simulink model "ADU_Integration_R2014a_simulation"  (R2014a)
settings: Solver=FixedStepDiscrete  StartTime=285  StopTime=300  FixedStep=0.01  RelTol=1e-3
PostLoadFcn:
  | , if any(exist('dsrtsu_mdlpostloadfcn', 'file') == [2, 3, 6]), try dsrtsu_mdlpostloadfcn('Execute', bdroot); catch fprintf('Error in PostLoadFcn (dsrtsu_mdlpostloadfcn) for model "%s":\n %s\n', bdroot, lasterr); end, end,
InitFcn:
  | load 'data/chi2_dat';
  | load 'data/Line_struct';
  | load 'data/innerLNM_1';
  | load 'data/middleLNM_2';
  | load 'data/outerLNM_1';
  | load 'data/landmarks_patac_schimmel_ccw';
  | load 'data/patac_navi_array';
  | load 'data/sensor';
  | load 'data/map_struct';
  | addpath map_src
  | Integration_Parameter;
  | load 'TestData_001';
values from neighbouring files (symbols this model uses):
  TestData_001 =     [TestData_001.mat]
undefined symbols (not defined in the file or in its folder): chi2_dat, innerLNM_1, landmarks_patac_schimmel_ccw, middleLNM_2, outerLNM_1, patac_navi_array
libraries: simulink x36, rtican x1
(part 4 of 22)

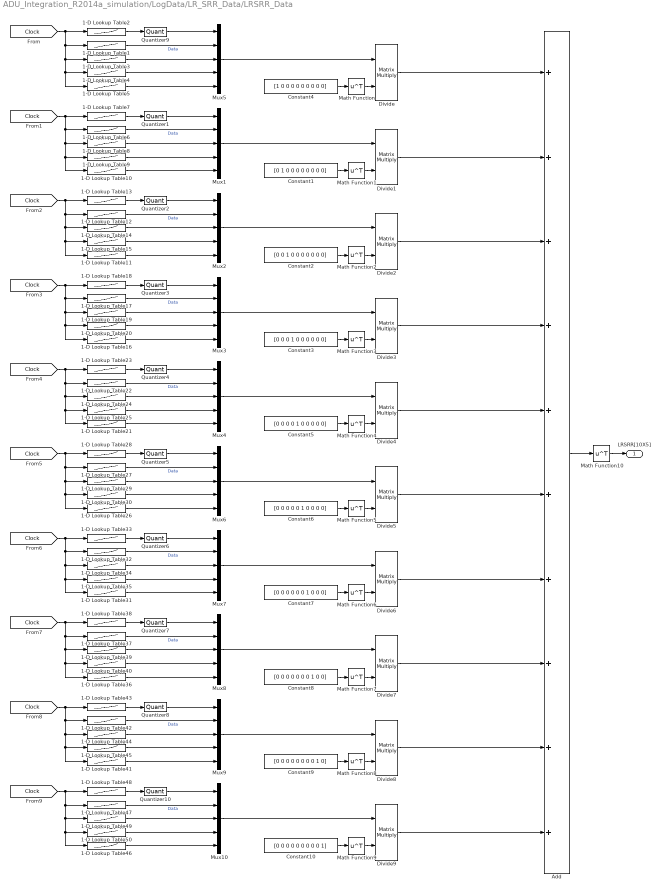
== system ADU_Integration_R2014a_simulation/LogData/LR_SRR_Data/LRSRR_Data ==
  1-D Lookup Table1 : Lookup_n-D  NumberOfTableDimensions=1  BreakpointsForDimension1=TestData_001.X.Data  Table=TestData_001.Y(StartNum+1+5*0).Data  RndMeth=Simplest  InputSameDT=on
  1-D Lookup Table10 : Lookup_n-D  NumberOfTableDimensions=1  BreakpointsForDimension1=TestData_001.X.Data  Table=TestData_001.Y(StartNum+4+5*1).Data  RndMeth=Simplest  InputSameDT=on
  1-D Lookup Table11 : Lookup_n-D  NumberOfTableDimensions=1  BreakpointsForDimension1=TestData_001.X.Data  Table=TestData_001.Y(StartNum+4+5*2).Data  RndMeth=Simplest  InputSameDT=on
  1-D Lookup Table12 : Lookup_n-D  NumberOfTableDimensions=1  BreakpointsForDimension1=TestData_001.X.Data  Table=TestData_001.Y(StartNum+1+5*2).Data  RndMeth=Simplest  InputSameDT=on
  1-D Lookup Table13 : Lookup_n-D  NumberOfTableDimensions=1  BreakpointsForDimension1=TestData_001.X.Data  Table=TestData_001.Y(StartNum+5*2).Data  RndMeth=Simplest  InputSameDT=on
  1-D Lookup Table14 : Lookup_n-D  NumberOfTableDimensions=1  BreakpointsForDimension1=TestData_001.X.Data  Table=TestData_001.Y(StartNum+2+5*2).Data  RndMeth=Simplest  InputSameDT=on
  1-D Lookup Table15 : Lookup_n-D  NumberOfTableDimensions=1  BreakpointsForDimension1=TestData_001.X.Data  Table=TestData_001.Y(StartNum+3+5*2).Data  RndMeth=Simplest  InputSameDT=on
  1-D Lookup Table16 : Lookup_n-D  NumberOfTableDimensions=1  BreakpointsForDimension1=TestData_001.X.Data  Table=TestData_001.Y(StartNum+4+5*3).Data  RndMeth=Simplest  InputSameDT=on
  1-D Lookup Table17 : Lookup_n-D  NumberOfTableDimensions=1  BreakpointsForDimension1=TestData_001.X.Data  Table=TestData_001.Y(StartNum+1+5*3).Data  RndMeth=Simplest  InputSameDT=on
  1-D Lookup Table18 : Lookup_n-D  NumberOfTableDimensions=1  BreakpointsForDimension1=TestData_001.X.Data  Table=TestData_001.Y(StartNum+5*3).Data  RndMeth=Simplest  InputSameDT=on
  1-D Lookup Table19 : Lookup_n-D  NumberOfTableDimensions=1  BreakpointsForDimension1=TestData_001.X.Data  Table=TestData_001.Y(StartNum+2+5*3).Data  RndMeth=Simplest  InputSameDT=on
  1-D Lookup Table2 : Lookup_n-D  NumberOfTableDimensions=1  BreakpointsForDimension1=TestData_001.X.Data  Table=TestData_001.Y(StartNum+5*0).Data  RndMeth=Simplest  InputSameDT=on
  1-D Lookup Table20 : Lookup_n-D  NumberOfTableDimensions=1  BreakpointsForDimension1=TestData_001.X.Data  Table=TestData_001.Y(StartNum+3+5*3).Data  RndMeth=Simplest  InputSameDT=on
  1-D Lookup Table21 : Lookup_n-D  NumberOfTableDimensions=1  BreakpointsForDimension1=TestData_001.X.Data  Table=TestData_001.Y(StartNum+4+5*4).Data  RndMeth=Simplest  InputSameDT=on
  1-D Lookup Table22 : Lookup_n-D  NumberOfTableDimensions=1  BreakpointsForDimension1=TestData_001.X.Data  Table=TestData_001.Y(StartNum+1+5*4).Data  RndMeth=Simplest  InputSameDT=on
  1-D Lookup Table23 : Lookup_n-D  NumberOfTableDimensions=1  BreakpointsForDimension1=TestData_001.X.Data  Table=TestData_001.Y(StartNum+5*4).Data  RndMeth=Simplest  InputSameDT=on
  1-D Lookup Table24 : Lookup_n-D  NumberOfTableDimensions=1  BreakpointsForDimension1=TestData_001.X.Data  Table=TestData_001.Y(StartNum+2+5*4).Data  RndMeth=Simplest  InputSameDT=on
  1-D Lookup Table25 : Lookup_n-D  NumberOfTableDimensions=1  BreakpointsForDimension1=TestData_001.X.Data  Table=TestData_001.Y(StartNum+3+5*4).Data  RndMeth=Simplest  InputSameDT=on
  1-D Lookup Table26 : Lookup_n-D  NumberOfTableDimensions=1  BreakpointsForDimension1=TestData_001.X.Data  Table=TestData_001.Y(StartNum+4+5*5).Data  RndMeth=Simplest  InputSameDT=on
  1-D Lookup Table27 : Lookup_n-D  NumberOfTableDimensions=1  BreakpointsForDimension1=TestData_001.X.Data  Table=TestData_001.Y(StartNum+1+5*5).Data  RndMeth=Simplest  InputSameDT=on
  1-D Lookup Table28 : Lookup_n-D  NumberOfTableDimensions=1  BreakpointsForDimension1=TestData_001.X.Data  Table=TestData_001.Y(StartNum+5*5).Data  RndMeth=Simplest  InputSameDT=on
  1-D Lookup Table29 : Lookup_n-D  NumberOfTableDimensions=1  BreakpointsForDimension1=TestData_001.X.Data  Table=TestData_001.Y(StartNum+2+5*5).Data  RndMeth=Simplest  InputSameDT=on
  1-D Lookup Table3 : Lookup_n-D  NumberOfTableDimensions=1  BreakpointsForDimension1=TestData_001.X.Data  Table=TestData_001.Y(StartNum+2+5*0).Data  RndMeth=Simplest  InputSameDT=on
  1-D Lookup Table30 : Lookup_n-D  NumberOfTableDimensions=1  BreakpointsForDimension1=TestData_001.X.Data  Table=TestData_001.Y(StartNum+3+5*5).Data  RndMeth=Simplest  InputSameDT=on
  1-D Lookup Table31 : Lookup_n-D  NumberOfTableDimensions=1  BreakpointsForDimension1=TestData_001.X.Data  Table=TestData_001.Y(StartNum+4+5*6).Data  RndMeth=Simplest  InputSameDT=on
  1-D Lookup Table32 : Lookup_n-D  NumberOfTableDimensions=1  BreakpointsForDimension1=TestData_001.X.Data  Table=TestData_001.Y(StartNum+1+5*6).Data  RndMeth=Simplest  InputSameDT=on
  1-D Lookup Table33 : Lookup_n-D  NumberOfTableDimensions=1  BreakpointsForDimension1=TestData_001.X.Data  Table=TestData_001.Y(StartNum+5*6).Data  RndMeth=Simplest  InputSameDT=on
  1-D Lookup Table34 : Lookup_n-D  NumberOfTableDimensions=1  BreakpointsForDimension1=TestData_001.X.Data  Table=TestData_001.Y(StartNum+2+5*6).Data  RndMeth=Simplest  InputSameDT=on
  1-D Lookup Table35 : Lookup_n-D  NumberOfTableDimensions=1  BreakpointsForDimension1=TestData_001.X.Data  Table=TestData_001.Y(StartNum+3+5*6).Data  RndMeth=Simplest  InputSameDT=on
  1-D Lookup Table36 : Lookup_n-D  NumberOfTableDimensions=1  BreakpointsForDimension1=TestData_001.X.Data  Table=TestData_001.Y(StartNum+4+5*7).Data  RndMeth=Simplest  InputSameDT=on
  1-D Lookup Table37 : Lookup_n-D  NumberOfTableDimensions=1  BreakpointsForDimension1=TestData_001.X.Data  Table=TestData_001.Y(StartNum+1+5*7).Data  RndMeth=Simplest  InputSameDT=on
  1-D Lookup Table38 : Lookup_n-D  NumberOfTableDimensions=1  BreakpointsForDimension1=TestData_001.X.Data  Table=TestData_001.Y(StartNum+5*7).Data  RndMeth=Simplest  InputSameDT=on
  1-D Lookup Table39 : Lookup_n-D  NumberOfTableDimensions=1  BreakpointsForDimension1=TestData_001.X.Data  Table=TestData_001.Y(StartNum+2+5*7).Data  RndMeth=Simplest  InputSameDT=on
  1-D Lookup Table4 : Lookup_n-D  NumberOfTableDimensions=1  BreakpointsForDimension1=TestData_001.X.Data  Table=TestData_001.Y(StartNum+3+5*0).Data  RndMeth=Simplest  InputSameDT=on
  1-D Lookup Table40 : Lookup_n-D  NumberOfTableDimensions=1  BreakpointsForDimension1=TestData_001.X.Data  Table=TestData_001.Y(StartNum+3+5*7).Data  RndMeth=Simplest  InputSameDT=on
  1-D Lookup Table41 : Lookup_n-D  NumberOfTableDimensions=1  BreakpointsForDimension1=TestData_001.X.Data  Table=TestData_001.Y(StartNum+4+5*8).Data  RndMeth=Simplest  InputSameDT=on
  1-D Lookup Table42 : Lookup_n-D  NumberOfTableDimensions=1  BreakpointsForDimension1=TestData_001.X.Data  Table=TestData_001.Y(StartNum+1+5*8).Data  RndMeth=Simplest  InputSameDT=on
  1-D Lookup Table43 : Lookup_n-D  NumberOfTableDimensions=1  BreakpointsForDimension1=TestData_001.X.Data  Table=TestData_001.Y(StartNum+5*8).Data  RndMeth=Simplest  InputSameDT=on
  1-D Lookup Table44 : Lookup_n-D  NumberOfTableDimensions=1  BreakpointsForDimension1=TestData_001.X.Data  Table=TestData_001.Y(StartNum+2+5*8).Data  RndMeth=Simplest  InputSameDT=on
  1-D Lookup Table45 : Lookup_n-D  NumberOfTableDimensions=1  BreakpointsForDimension1=TestData_001.X.Data  Table=TestData_001.Y(StartNum+3+5*8).Data  RndMeth=Simplest  InputSameDT=on
  1-D Lookup Table46 : Lookup_n-D  NumberOfTableDimensions=1  BreakpointsForDimension1=TestData_001.X.Data  Table=TestData_001.Y(StartNum+4+5*9).Data  RndMeth=Simplest  InputSameDT=on
  1-D Lookup Table47 : Lookup_n-D  NumberOfTableDimensions=1  BreakpointsForDimension1=TestData_001.X.Data  Table=TestData_001.Y(StartNum+1+5*9).Data  RndMeth=Simplest  InputSameDT=on
  1-D Lookup Table48 : Lookup_n-D  NumberOfTableDimensions=1  BreakpointsForDimension1=TestData_001.X.Data  Table=TestData_001.Y(StartNum+5*9).Data  RndMeth=Simplest  InputSameDT=on
  1-D Lookup Table49 : Lookup_n-D  NumberOfTableDimensions=1  BreakpointsForDimension1=TestData_001.X.Data  Table=TestData_001.Y(StartNum+2+5*9).Data  RndMeth=Simplest  InputSameDT=on
  1-D Lookup Table5 : Lookup_n-D  NumberOfTableDimensions=1  BreakpointsForDimension1=TestData_001.X.Data  Table=TestData_001.Y(StartNum+4+5*0).Data  RndMeth=Simplest  InputSameDT=on
  1-D Lookup Table50 : Lookup_n-D  NumberOfTableDimensions=1  BreakpointsForDimension1=TestData_001.X.Data  Table=TestData_001.Y(StartNum+3+5*9).Data  RndMeth=Simplest  InputSameDT=on
  1-D Lookup Table6 : Lookup_n-D  NumberOfTableDimensions=1  BreakpointsForDimension1=TestData_001.X.Data  Table=TestData_001.Y(StartNum+1+5*1).Data  RndMeth=Simplest  InputSameDT=on
  1-D Lookup Table7 : Lookup_n-D  NumberOfTableDimensions=1  BreakpointsForDimension1=TestData_001.X.Data  Table=TestData_001.Y(StartNum+5*1).Data  RndMeth=Simplest  InputSameDT=on
  1-D Lookup Table8 : Lookup_n-D  NumberOfTableDimensions=1  BreakpointsForDimension1=TestData_001.X.Data  Table=TestData_001.Y(StartNum+2+5*1).Data  RndMeth=Simplest  InputSameDT=on
  1-D Lookup Table9 : Lookup_n-D  NumberOfTableDimensions=1  BreakpointsForDimension1=TestData_001.X.Data  Table=TestData_001.Y(StartNum+3+5*1).Data  RndMeth=Simplest  InputSameDT=on
  Add : Sum  Inputs=++++++++++
  Constant1 : Constant  Value=[0 1 0 0 0 0 0 0 0 0]
  Constant10 : Constant  Value=[0 0 0 0 0 0 0 0 0 1]
  Constant2 : Constant  Value=[0 0 1 0 0 0 0 0 0 0]
  Constant3 : Constant  Value=[0 0 0 1 0 0 0 0 0 0]
  Constant4 : Constant  Value=[1 0 0 0 0 0 0 0 0 0]
  Constant5 : Constant  Value=[0 0 0 0 1 0 0 0 0 0]
  Constant6 : Constant  Value=[0 0 0 0 0 1 0 0 0 0]
  Constant7 : Constant  Value=[0 0 0 0 0 0 1 0 0 0]
  Constant8 : Constant  Value=[0 0 0 0 0 0 0 1 0 0]
  Constant9 : Constant  Value=[0 0 0 0 0 0 0 0 1 0]
  Divide{,1..9} (10 alike) : Product  Inputs=**  Multiplication=Matrix(*)
  Math Function{,1..10} (11 alike) : Math  Operator=transpose  SaturateOnIntegerOverflow=on
  Mux{1..10} (10 alike) : Mux  Inputs=5
  Quantizer{1..10} (10 alike) : Quantizer  QuantizationInterval=1
  LRSRR[10X5] : Outport
  wires:
  Mux5/1 -> Divide/1
  Constant4/1 -> Math Function/1
  Math Function/1 -> Divide/2
  Divide/1 -> Add/1
  Math Function4/1 -> Divide4/2
  Math Function3/1 -> Divide3/2
  Divide3/1 -> Add/4
  Constant9/1 -> Math Function8/1
  Math Function6/1 -> Divide6/2
  Divide1/1 -> Add/2
  Divide4/1 -> Add/5
  Quantizer9/1 -> Mux5/1
  Constant7/1 -> Math Function6/1
  Divide2/1 -> Add/3
  Divide9/1 -> Add/10
  Constant3/1 -> Math Function3/1
  Divide5/1 -> Add/6
  Math Function5/1 -> Divide5/2
  1-D Lookup Table4/1 -> Mux5/4
  1-D Lookup Table3/1 -> Mux5/3
  Constant8/1 -> Math Function7/1
  Divide6/1 -> Add/7
  Math Function8/1 -> Divide8/2
  Constant5/1 -> Math Function4/1
  Math Function9/1 -> Divide9/2
  Math Function7/1 -> Divide7/2
  Constant10/1 -> Math Function9/1
  Math Function2/1 -> Divide2/2
  Constant1/1 -> Math Function1/1
  Divide7/1 -> Add/8
  Divide8/1 -> Add/9
  Constant2/1 -> Math Function2/1
  Math Function1/1 -> Divide1/2
  Constant6/1 -> Math Function5/1
  Add/1 -> Math Function10/1
  Math Function10/1 -> LRSRR[10X5]/1
  1-D Lookup Table2/1 -> Quantizer9/1
  [Clock] -> 1-D Lookup Table2/1, 1-D Lookup Table1/1, 1-D Lookup Table5/1, 1-D Lookup Table4/1, 1-D Lookup Table3/1
  1-D Lookup Table1/1 -> Mux5/2  "Data"
  1-D Lookup Table5/1 -> Mux5/5
  Mux1/1 -> Divide1/1
  Quantizer1/1 -> Mux1/1
  1-D Lookup Table9/1 -> Mux1/4
  1-D Lookup Table8/1 -> Mux1/3
  1-D Lookup Table7/1 -> Quantizer1/1
  [Clock] -> 1-D Lookup Table7/1, 1-D Lookup Table6/1, 1-D Lookup Table8/1, 1-D Lookup Table10/1, 1-D Lookup Table9/1
  1-D Lookup Table6/1 -> Mux1/2  "Data"
  1-D Lookup Table10/1 -> Mux1/5
  Mux2/1 -> Divide2/1
  Quantizer2/1 -> Mux2/1
  1-D Lookup Table15/1 -> Mux2/4
  1-D Lookup Table14/1 -> Mux2/3
  1-D Lookup Table13/1 -> Quantizer2/1
  [Clock] -> 1-D Lookup Table13/1, 1-D Lookup Table12/1, 1-D Lookup Table14/1, 1-D Lookup Table15/1, 1-D Lookup Table11/1
  1-D Lookup Table12/1 -> Mux2/2  "Data"
  1-D Lookup Table11/1 -> Mux2/5
  Mux3/1 -> Divide3/1
  Quantizer3/1 -> Mux3/1
  1-D Lookup Table20/1 -> Mux3/4
  1-D Lookup Table19/1 -> Mux3/3
  1-D Lookup Table18/1 -> Quantizer3/1
  [Clock] -> 1-D Lookup Table18/1, 1-D Lookup Table17/1, 1-D Lookup Table19/1, 1-D Lookup Table20/1, 1-D Lookup Table16/1
  1-D Lookup Table17/1 -> Mux3/2  "Data"
  1-D Lookup Table16/1 -> Mux3/5
  Mux4/1 -> Divide4/1
  Quantizer4/1 -> Mux4/1
  1-D Lookup Table25/1 -> Mux4/4
  1-D Lookup Table24/1 -> Mux4/3
  1-D Lookup Table23/1 -> Quantizer4/1
  [Clock] -> 1-D Lookup Table23/1, 1-D Lookup Table22/1, 1-D Lookup Table24/1, 1-D Lookup Table21/1, 1-D Lookup Table25/1
  1-D Lookup Table22/1 -> Mux4/2  "Data"
  1-D Lookup Table21/1 -> Mux4/5
  Mux6/1 -> Divide5/1
  Quantizer5/1 -> Mux6/1
  1-D Lookup Table30/1 -> Mux6/4
  1-D Lookup Table29/1 -> Mux6/3
  1-D Lookup Table28/1 -> Quantizer5/1
  [Clock] -> 1-D Lookup Table28/1, 1-D Lookup Table27/1, 1-D Lookup Table29/1, 1-D Lookup Table30/1, 1-D Lookup Table26/1
  1-D Lookup Table27/1 -> Mux6/2  "Data"
  1-D Lookup Table26/1 -> Mux6/5
  Mux7/1 -> Divide6/1
  Quantizer6/1 -> Mux7/1
  1-D Lookup Table35/1 -> Mux7/4
  1-D Lookup Table34/1 -> Mux7/3
  1-D Lookup Table33/1 -> Quantizer6/1
  [Clock] -> 1-D Lookup Table33/1, 1-D Lookup Table32/1, 1-D Lookup Table34/1, 1-D Lookup Table31/1, 1-D Lookup Table35/1
  1-D Lookup Table32/1 -> Mux7/2  "Data"
  1-D Lookup Table31/1 -> Mux7/5
  Mux8/1 -> Divide7/1
  Quantizer7/1 -> Mux8/1
  1-D Lookup Table40/1 -> Mux8/4
  1-D Lookup Table39/1 -> Mux8/3
  1-D Lookup Table38/1 -> Quantizer7/1
  [Clock] -> 1-D Lookup Table38/1, 1-D Lookup Table37/1, 1-D Lookup Table39/1, 1-D Lookup Table40/1, 1-D Lookup Table36/1
  1-D Lookup Table37/1 -> Mux8/2  "Data"
  1-D Lookup Table36/1 -> Mux8/5
  Mux9/1 -> Divide8/1
  Quantizer8/1 -> Mux9/1
  1-D Lookup Table45/1 -> Mux9/4
  1-D Lookup Table44/1 -> Mux9/3
  1-D Lookup Table43/1 -> Quantizer8/1
  [Clock] -> 1-D Lookup Table43/1, 1-D Lookup Table42/1, 1-D Lookup Table44/1, 1-D Lookup Table41/1, 1-D Lookup Table45/1
  1-D Lookup Table42/1 -> Mux9/2  "Data"
  1-D Lookup Table41/1 -> Mux9/5
  Mux10/1 -> Divide9/1
  Quantizer10/1 -> Mux10/1
  1-D Lookup Table50/1 -> Mux10/4
  1-D Lookup Table49/1 -> Mux10/3
  1-D Lookup Table48/1 -> Quantizer10/1
  [Clock] -> 1-D Lookup Table48/1, 1-D Lookup Table47/1, 1-D Lookup Table49/1, 1-D Lookup Table50/1, 1-D Lookup Table46/1
  1-D Lookup Table47/1 -> Mux10/2  "Data"
  1-D Lookup Table46/1 -> Mux10/5

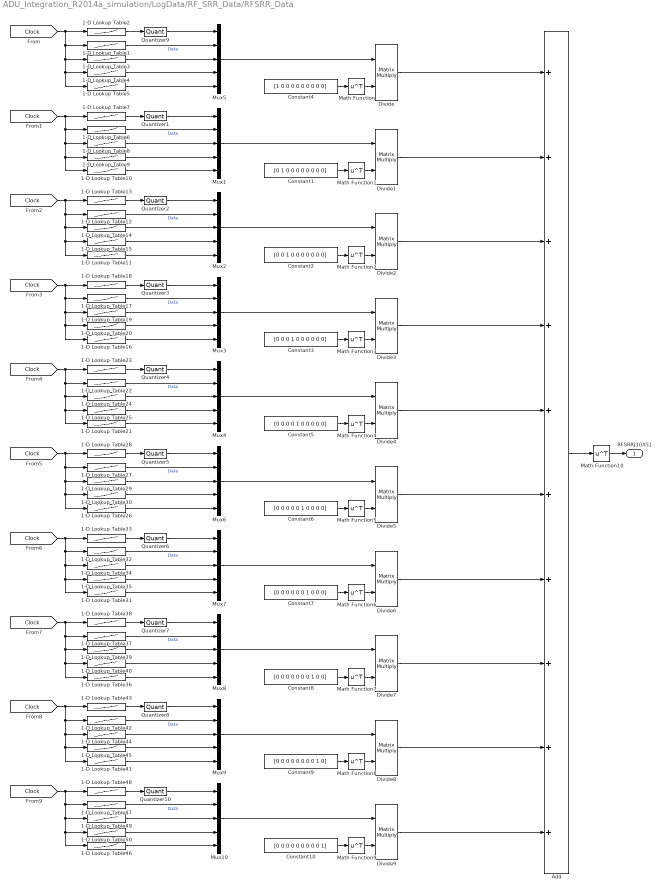
== system ADU_Integration_R2014a_simulation/LogData/RF_SRR_Data/RFSRR_Data ==
  1-D Lookup Table1 : Lookup_n-D  NumberOfTableDimensions=1  BreakpointsForDimension1=TestData_001.X.Data  Table=TestData_001.Y(StartNum+1+5*0).Data  RndMeth=Simplest  InputSameDT=on
  1-D Lookup Table10 : Lookup_n-D  NumberOfTableDimensions=1  BreakpointsForDimension1=TestData_001.X.Data  Table=TestData_001.Y(StartNum+4+5*1).Data  RndMeth=Simplest  InputSameDT=on
  1-D Lookup Table11 : Lookup_n-D  NumberOfTableDimensions=1  BreakpointsForDimension1=TestData_001.X.Data  Table=TestData_001.Y(StartNum+4+5*2).Data  RndMeth=Simplest  InputSameDT=on
  1-D Lookup Table12 : Lookup_n-D  NumberOfTableDimensions=1  BreakpointsForDimension1=TestData_001.X.Data  Table=TestData_001.Y(StartNum+1+5*2).Data  RndMeth=Simplest  InputSameDT=on
  1-D Lookup Table13 : Lookup_n-D  NumberOfTableDimensions=1  BreakpointsForDimension1=TestData_001.X.Data  Table=TestData_001.Y(StartNum+5*2).Data  RndMeth=Simplest  InputSameDT=on
  1-D Lookup Table14 : Lookup_n-D  NumberOfTableDimensions=1  BreakpointsForDimension1=TestData_001.X.Data  Table=TestData_001.Y(StartNum+2+5*2).Data  RndMeth=Simplest  InputSameDT=on
  1-D Lookup Table15 : Lookup_n-D  NumberOfTableDimensions=1  BreakpointsForDimension1=TestData_001.X.Data  Table=TestData_001.Y(StartNum+3+5*2).Data  RndMeth=Simplest  InputSameDT=on
  1-D Lookup Table16 : Lookup_n-D  NumberOfTableDimensions=1  BreakpointsForDimension1=TestData_001.X.Data  Table=TestData_001.Y(StartNum+4+5*3).Data  RndMeth=Simplest  InputSameDT=on
  1-D Lookup Table17 : Lookup_n-D  NumberOfTableDimensions=1  BreakpointsForDimension1=TestData_001.X.Data  Table=TestData_001.Y(StartNum+1+5*3).Data  RndMeth=Simplest  InputSameDT=on
  1-D Lookup Table18 : Lookup_n-D  NumberOfTableDimensions=1  BreakpointsForDimension1=TestData_001.X.Data  Table=TestData_001.Y(StartNum+5*3).Data  RndMeth=Simplest  InputSameDT=on
  1-D Lookup Table19 : Lookup_n-D  NumberOfTableDimensions=1  BreakpointsForDimension1=TestData_001.X.Data  Table=TestData_001.Y(StartNum+2+5*3).Data  RndMeth=Simplest  InputSameDT=on
  1-D Lookup Table2 : Lookup_n-D  NumberOfTableDimensions=1  BreakpointsForDimension1=TestData_001.X.Data  Table=TestData_001.Y(StartNum+5*0).Data  RndMeth=Simplest  InputSameDT=on
  1-D Lookup Table20 : Lookup_n-D  NumberOfTableDimensions=1  BreakpointsForDimension1=TestData_001.X.Data  Table=TestData_001.Y(StartNum+3+5*3).Data  RndMeth=Simplest  InputSameDT=on
  1-D Lookup Table21 : Lookup_n-D  NumberOfTableDimensions=1  BreakpointsForDimension1=TestData_001.X.Data  Table=TestData_001.Y(StartNum+4+5*4).Data  RndMeth=Simplest  InputSameDT=on
  1-D Lookup Table22 : Lookup_n-D  NumberOfTableDimensions=1  BreakpointsForDimension1=TestData_001.X.Data  Table=TestData_001.Y(StartNum+1+5*4).Data  RndMeth=Simplest  InputSameDT=on
  1-D Lookup Table23 : Lookup_n-D  NumberOfTableDimensions=1  BreakpointsForDimension1=TestData_001.X.Data  Table=TestData_001.Y(StartNum+5*4).Data  RndMeth=Simplest  InputSameDT=on
  1-D Lookup Table24 : Lookup_n-D  NumberOfTableDimensions=1  BreakpointsForDimension1=TestData_001.X.Data  Table=TestData_001.Y(StartNum+2+5*4).Data  RndMeth=Simplest  InputSameDT=on
  1-D Lookup Table25 : Lookup_n-D  NumberOfTableDimensions=1  BreakpointsForDimension1=TestData_001.X.Data  Table=TestData_001.Y(StartNum+3+5*4).Data  RndMeth=Simplest  InputSameDT=on
  1-D Lookup Table26 : Lookup_n-D  NumberOfTableDimensions=1  BreakpointsForDimension1=TestData_001.X.Data  Table=TestData_001.Y(StartNum+4+5*5).Data  RndMeth=Simplest  InputSameDT=on
  1-D Lookup Table27 : Lookup_n-D  NumberOfTableDimensions=1  BreakpointsForDimension1=TestData_001.X.Data  Table=TestData_001.Y(StartNum+1+5*5).Data  RndMeth=Simplest  InputSameDT=on
  1-D Lookup Table28 : Lookup_n-D  NumberOfTableDimensions=1  BreakpointsForDimension1=TestData_001.X.Data  Table=TestData_001.Y(StartNum+5*5).Data  RndMeth=Simplest  InputSameDT=on
  1-D Lookup Table29 : Lookup_n-D  NumberOfTableDimensions=1  BreakpointsForDimension1=TestData_001.X.Data  Table=TestData_001.Y(StartNum+2+5*5).Data  RndMeth=Simplest  InputSameDT=on
  1-D Lookup Table3 : Lookup_n-D  NumberOfTableDimensions=1  BreakpointsForDimension1=TestData_001.X.Data  Table=TestData_001.Y(StartNum+2+5*0).Data  RndMeth=Simplest  InputSameDT=on
  1-D Lookup Table30 : Lookup_n-D  NumberOfTableDimensions=1  BreakpointsForDimension1=TestData_001.X.Data  Table=TestData_001.Y(StartNum+3+5*5).Data  RndMeth=Simplest  InputSameDT=on
  1-D Lookup Table31 : Lookup_n-D  NumberOfTableDimensions=1  BreakpointsForDimension1=TestData_001.X.Data  Table=TestData_001.Y(StartNum+4+5*6).Data  RndMeth=Simplest  InputSameDT=on
  1-D Lookup Table32 : Lookup_n-D  NumberOfTableDimensions=1  BreakpointsForDimension1=TestData_001.X.Data  Table=TestData_001.Y(StartNum+1+5*6).Data  RndMeth=Simplest  InputSameDT=on
  1-D Lookup Table33 : Lookup_n-D  NumberOfTableDimensions=1  BreakpointsForDimension1=TestData_001.X.Data  Table=TestData_001.Y(StartNum+5*6).Data  RndMeth=Simplest  InputSameDT=on
  1-D Lookup Table34 : Lookup_n-D  NumberOfTableDimensions=1  BreakpointsForDimension1=TestData_001.X.Data  Table=TestData_001.Y(StartNum+2+5*6).Data  RndMeth=Simplest  InputSameDT=on
  1-D Lookup Table35 : Lookup_n-D  NumberOfTableDimensions=1  BreakpointsForDimension1=TestData_001.X.Data  Table=TestData_001.Y(StartNum+3+5*6).Data  RndMeth=Simplest  InputSameDT=on
  1-D Lookup Table36 : Lookup_n-D  NumberOfTableDimensions=1  BreakpointsForDimension1=TestData_001.X.Data  Table=TestData_001.Y(StartNum+4+5*7).Data  RndMeth=Simplest  InputSameDT=on
  1-D Lookup Table37 : Lookup_n-D  NumberOfTableDimensions=1  BreakpointsForDimension1=TestData_001.X.Data  Table=TestData_001.Y(StartNum+1+5*7).Data  RndMeth=Simplest  InputSameDT=on
  1-D Lookup Table38 : Lookup_n-D  NumberOfTableDimensions=1  BreakpointsForDimension1=TestData_001.X.Data  Table=TestData_001.Y(StartNum+5*7).Data  RndMeth=Simplest  InputSameDT=on
  1-D Lookup Table39 : Lookup_n-D  NumberOfTableDimensions=1  BreakpointsForDimension1=TestData_001.X.Data  Table=TestData_001.Y(StartNum+2+5*7).Data  RndMeth=Simplest  InputSameDT=on
  1-D Lookup Table4 : Lookup_n-D  NumberOfTableDimensions=1  BreakpointsForDimension1=TestData_001.X.Data  Table=TestData_001.Y(StartNum+3+5*0).Data  RndMeth=Simplest  InputSameDT=on
  1-D Lookup Table40 : Lookup_n-D  NumberOfTableDimensions=1  BreakpointsForDimension1=TestData_001.X.Data  Table=TestData_001.Y(StartNum+3+5*7).Data  RndMeth=Simplest  InputSameDT=on
  1-D Lookup Table41 : Lookup_n-D  NumberOfTableDimensions=1  BreakpointsForDimension1=TestData_001.X.Data  Table=TestData_001.Y(StartNum+4+5*8).Data  RndMeth=Simplest  InputSameDT=on
  1-D Lookup Table42 : Lookup_n-D  NumberOfTableDimensions=1  BreakpointsForDimension1=TestData_001.X.Data  Table=TestData_001.Y(StartNum+1+5*8).Data  RndMeth=Simplest  InputSameDT=on
  1-D Lookup Table43 : Lookup_n-D  NumberOfTableDimensions=1  BreakpointsForDimension1=TestData_001.X.Data  Table=TestData_001.Y(StartNum+5*8).Data  RndMeth=Simplest  InputSameDT=on
  1-D Lookup Table44 : Lookup_n-D  NumberOfTableDimensions=1  BreakpointsForDimension1=TestData_001.X.Data  Table=TestData_001.Y(StartNum+2+5*8).Data  RndMeth=Simplest  InputSameDT=on
  1-D Lookup Table45 : Lookup_n-D  NumberOfTableDimensions=1  BreakpointsForDimension1=TestData_001.X.Data  Table=TestData_001.Y(StartNum+3+5*8).Data  RndMeth=Simplest  InputSameDT=on
  1-D Lookup Table46 : Lookup_n-D  NumberOfTableDimensions=1  BreakpointsForDimension1=TestData_001.X.Data  Table=TestData_001.Y(StartNum+4+5*9).Data  RndMeth=Simplest  InputSameDT=on
  1-D Lookup Table47 : Lookup_n-D  NumberOfTableDimensions=1  BreakpointsForDimension1=TestData_001.X.Data  Table=TestData_001.Y(StartNum+1+5*9).Data  RndMeth=Simplest  InputSameDT=on
  1-D Lookup Table48 : Lookup_n-D  NumberOfTableDimensions=1  BreakpointsForDimension1=TestData_001.X.Data  Table=TestData_001.Y(StartNum+5*9).Data  RndMeth=Simplest  InputSameDT=on
  1-D Lookup Table49 : Lookup_n-D  NumberOfTableDimensions=1  BreakpointsForDimension1=TestData_001.X.Data  Table=TestData_001.Y(StartNum+2+5*9).Data  RndMeth=Simplest  InputSameDT=on
  1-D Lookup Table5 : Lookup_n-D  NumberOfTableDimensions=1  BreakpointsForDimension1=TestData_001.X.Data  Table=TestData_001.Y(StartNum+4+5*0).Data  RndMeth=Simplest  InputSameDT=on
  1-D Lookup Table50 : Lookup_n-D  NumberOfTableDimensions=1  BreakpointsForDimension1=TestData_001.X.Data  Table=TestData_001.Y(StartNum+3+5*9).Data  RndMeth=Simplest  InputSameDT=on
  1-D Lookup Table6 : Lookup_n-D  NumberOfTableDimensions=1  BreakpointsForDimension1=TestData_001.X.Data  Table=TestData_001.Y(StartNum+1+5*1).Data  RndMeth=Simplest  InputSameDT=on
  1-D Lookup Table7 : Lookup_n-D  NumberOfTableDimensions=1  BreakpointsForDimension1=TestData_001.X.Data  Table=TestData_001.Y(StartNum+5*1).Data  RndMeth=Simplest  InputSameDT=on
  1-D Lookup Table8 : Lookup_n-D  NumberOfTableDimensions=1  BreakpointsForDimension1=TestData_001.X.Data  Table=TestData_001.Y(StartNum+2+5*1).Data  RndMeth=Simplest  InputSameDT=on
  1-D Lookup Table9 : Lookup_n-D  NumberOfTableDimensions=1  BreakpointsForDimension1=TestData_001.X.Data  Table=TestData_001.Y(StartNum+3+5*1).Data  RndMeth=Simplest  InputSameDT=on
  Add : Sum  Inputs=++++++++++
  Constant1 : Constant  Value=[0 1 0 0 0 0 0 0 0 0]
  Constant10 : Constant  Value=[0 0 0 0 0 0 0 0 0 1]
  Constant2 : Constant  Value=[0 0 1 0 0 0 0 0 0 0]
  Constant3 : Constant  Value=[0 0 0 1 0 0 0 0 0 0]
  Constant4 : Constant  Value=[1 0 0 0 0 0 0 0 0 0]
  Constant5 : Constant  Value=[0 0 0 0 1 0 0 0 0 0]
  Constant6 : Constant  Value=[0 0 0 0 0 1 0 0 0 0]
  Constant7 : Constant  Value=[0 0 0 0 0 0 1 0 0 0]
  Constant8 : Constant  Value=[0 0 0 0 0 0 0 1 0 0]
  Constant9 : Constant  Value=[0 0 0 0 0 0 0 0 1 0]
  Divide{,1..9} (10 alike) : Product  Inputs=**  Multiplication=Matrix(*)
  Math Function{,1..10} (11 alike) : Math  Operator=transpose  SaturateOnIntegerOverflow=on
  Mux{1..10} (10 alike) : Mux  Inputs=5
  Quantizer{1..10} (10 alike) : Quantizer  QuantizationInterval=1
  RFSRR[10X5] : Outport
  wires:
  Mux5/1 -> Divide/1
  Constant4/1 -> Math Function/1
  Math Function/1 -> Divide/2
  Divide/1 -> Add/1
  Math Function4/1 -> Divide4/2
  Math Function3/1 -> Divide3/2
  Divide3/1 -> Add/4
  Constant9/1 -> Math Function8/1
  Math Function6/1 -> Divide6/2
  Divide1/1 -> Add/2
  Divide4/1 -> Add/5
  Quantizer9/1 -> Mux5/1
  Constant7/1 -> Math Function6/1
  Divide2/1 -> Add/3
  Divide9/1 -> Add/10
  Constant3/1 -> Math Function3/1
  Divide5/1 -> Add/6
  Math Function5/1 -> Divide5/2
  1-D Lookup Table4/1 -> Mux5/4
  1-D Lookup Table3/1 -> Mux5/3
  Constant8/1 -> Math Function7/1
  Divide6/1 -> Add/7
  Math Function8/1 -> Divide8/2
  Constant5/1 -> Math Function4/1
  Math Function9/1 -> Divide9/2
  Math Function7/1 -> Divide7/2
  Constant10/1 -> Math Function9/1
  Math Function2/1 -> Divide2/2
  Constant1/1 -> Math Function1/1
  Divide7/1 -> Add/8
  Divide8/1 -> Add/9
  Constant2/1 -> Math Function2/1
  Math Function1/1 -> Divide1/2
  Constant6/1 -> Math Function5/1
  Add/1 -> Math Function10/1
  Math Function10/1 -> RFSRR[10X5]/1
  1-D Lookup Table2/1 -> Quantizer9/1
  [Clock] -> 1-D Lookup Table2/1, 1-D Lookup Table1/1, 1-D Lookup Table5/1, 1-D Lookup Table4/1, 1-D Lookup Table3/1
  1-D Lookup Table1/1 -> Mux5/2  "Data"
  1-D Lookup Table5/1 -> Mux5/5
  Mux1/1 -> Divide1/1
  Quantizer1/1 -> Mux1/1
  1-D Lookup Table9/1 -> Mux1/4
  1-D Lookup Table8/1 -> Mux1/3
  1-D Lookup Table7/1 -> Quantizer1/1
  [Clock] -> 1-D Lookup Table7/1, 1-D Lookup Table6/1, 1-D Lookup Table8/1, 1-D Lookup Table10/1, 1-D Lookup Table9/1
  1-D Lookup Table6/1 -> Mux1/2  "Data"
  1-D Lookup Table10/1 -> Mux1/5
  Mux2/1 -> Divide2/1
  Quantizer2/1 -> Mux2/1
  1-D Lookup Table15/1 -> Mux2/4
  1-D Lookup Table14/1 -> Mux2/3
  1-D Lookup Table13/1 -> Quantizer2/1
  [Clock] -> 1-D Lookup Table13/1, 1-D Lookup Table12/1, 1-D Lookup Table14/1, 1-D Lookup Table15/1, 1-D Lookup Table11/1
  1-D Lookup Table12/1 -> Mux2/2  "Data"
  1-D Lookup Table11/1 -> Mux2/5
  Mux3/1 -> Divide3/1
  Quantizer3/1 -> Mux3/1
  1-D Lookup Table20/1 -> Mux3/4
  1-D Lookup Table19/1 -> Mux3/3
  1-D Lookup Table18/1 -> Quantizer3/1
  [Clock] -> 1-D Lookup Table18/1, 1-D Lookup Table17/1, 1-D Lookup Table19/1, 1-D Lookup Table20/1, 1-D Lookup Table16/1
  1-D Lookup Table17/1 -> Mux3/2  "Data"
  1-D Lookup Table16/1 -> Mux3/5
  Mux4/1 -> Divide4/1
  Quantizer4/1 -> Mux4/1
  1-D Lookup Table25/1 -> Mux4/4
  1-D Lookup Table24/1 -> Mux4/3
  1-D Lookup Table23/1 -> Quantizer4/1
  [Clock] -> 1-D Lookup Table23/1, 1-D Lookup Table22/1, 1-D Lookup Table24/1, 1-D Lookup Table21/1, 1-D Lookup Table25/1
  1-D Lookup Table22/1 -> Mux4/2  "Data"
  1-D Lookup Table21/1 -> Mux4/5
  Mux6/1 -> Divide5/1
  Quantizer5/1 -> Mux6/1
  1-D Lookup Table30/1 -> Mux6/4
  1-D Lookup Table29/1 -> Mux6/3
  1-D Lookup Table28/1 -> Quantizer5/1
  [Clock] -> 1-D Lookup Table28/1, 1-D Lookup Table27/1, 1-D Lookup Table29/1, 1-D Lookup Table30/1, 1-D Lookup Table26/1
  1-D Lookup Table27/1 -> Mux6/2  "Data"
  1-D Lookup Table26/1 -> Mux6/5
  Mux7/1 -> Divide6/1
  Quantizer6/1 -> Mux7/1
  1-D Lookup Table35/1 -> Mux7/4
  1-D Lookup Table34/1 -> Mux7/3
  1-D Lookup Table33/1 -> Quantizer6/1
  [Clock] -> 1-D Lookup Table33/1, 1-D Lookup Table32/1, 1-D Lookup Table34/1, 1-D Lookup Table31/1, 1-D Lookup Table35/1
  1-D Lookup Table32/1 -> Mux7/2  "Data"
  1-D Lookup Table31/1 -> Mux7/5
  Mux8/1 -> Divide7/1
  Quantizer7/1 -> Mux8/1
  1-D Lookup Table40/1 -> Mux8/4
  1-D Lookup Table39/1 -> Mux8/3
  1-D Lookup Table38/1 -> Quantizer7/1
  [Clock] -> 1-D Lookup Table38/1, 1-D Lookup Table37/1, 1-D Lookup Table39/1, 1-D Lookup Table40/1, 1-D Lookup Table36/1
  1-D Lookup Table37/1 -> Mux8/2  "Data"
  1-D Lookup Table36/1 -> Mux8/5
  Mux9/1 -> Divide8/1
  Quantizer8/1 -> Mux9/1
  1-D Lookup Table45/1 -> Mux9/4
  1-D Lookup Table44/1 -> Mux9/3
  1-D Lookup Table43/1 -> Quantizer8/1
  [Clock] -> 1-D Lookup Table43/1, 1-D Lookup Table42/1, 1-D Lookup Table44/1, 1-D Lookup Table41/1, 1-D Lookup Table45/1
  1-D Lookup Table42/1 -> Mux9/2  "Data"
  1-D Lookup Table41/1 -> Mux9/5
  Mux10/1 -> Divide9/1
  Quantizer10/1 -> Mux10/1
  1-D Lookup Table50/1 -> Mux10/4
  1-D Lookup Table49/1 -> Mux10/3
  1-D Lookup Table48/1 -> Quantizer10/1
  [Clock] -> 1-D Lookup Table48/1, 1-D Lookup Table47/1, 1-D Lookup Table49/1, 1-D Lookup Table50/1, 1-D Lookup Table46/1
  1-D Lookup Table47/1 -> Mux10/2  "Data"
  1-D Lookup Table46/1 -> Mux10/5

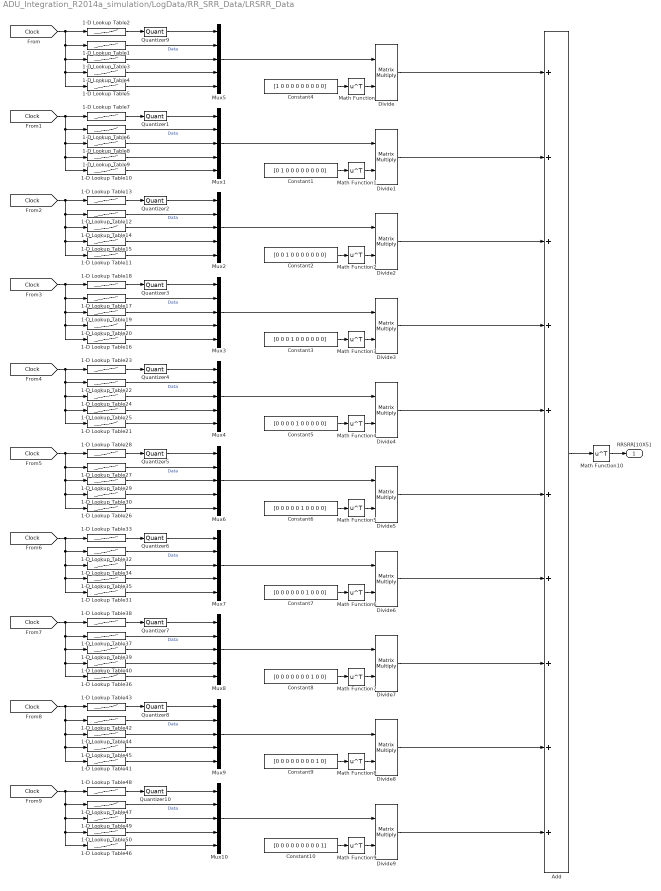
== system ADU_Integration_R2014a_simulation/LogData/RR_SRR_Data/LRSRR_Data ==
  1-D Lookup Table1 : Lookup_n-D  NumberOfTableDimensions=1  BreakpointsForDimension1=TestData_001.X.Data  Table=TestData_001.Y(StartNum+1+5*0).Data  RndMeth=Simplest  InputSameDT=on
  1-D Lookup Table10 : Lookup_n-D  NumberOfTableDimensions=1  BreakpointsForDimension1=TestData_001.X.Data  Table=TestData_001.Y(StartNum+4+5*1).Data  RndMeth=Simplest  InputSameDT=on
  1-D Lookup Table11 : Lookup_n-D  NumberOfTableDimensions=1  BreakpointsForDimension1=TestData_001.X.Data  Table=TestData_001.Y(StartNum+4+5*2).Data  RndMeth=Simplest  InputSameDT=on
  1-D Lookup Table12 : Lookup_n-D  NumberOfTableDimensions=1  BreakpointsForDimension1=TestData_001.X.Data  Table=TestData_001.Y(StartNum+1+5*2).Data  RndMeth=Simplest  InputSameDT=on
  1-D Lookup Table13 : Lookup_n-D  NumberOfTableDimensions=1  BreakpointsForDimension1=TestData_001.X.Data  Table=TestData_001.Y(StartNum+5*2).Data  RndMeth=Simplest  InputSameDT=on
  1-D Lookup Table14 : Lookup_n-D  NumberOfTableDimensions=1  BreakpointsForDimension1=TestData_001.X.Data  Table=TestData_001.Y(StartNum+2+5*2).Data  RndMeth=Simplest  InputSameDT=on
  1-D Lookup Table15 : Lookup_n-D  NumberOfTableDimensions=1  BreakpointsForDimension1=TestData_001.X.Data  Table=TestData_001.Y(StartNum+3+5*2).Data  RndMeth=Simplest  InputSameDT=on
  1-D Lookup Table16 : Lookup_n-D  NumberOfTableDimensions=1  BreakpointsForDimension1=TestData_001.X.Data  Table=TestData_001.Y(StartNum+4+5*3).Data  RndMeth=Simplest  InputSameDT=on
  1-D Lookup Table17 : Lookup_n-D  NumberOfTableDimensions=1  BreakpointsForDimension1=TestData_001.X.Data  Table=TestData_001.Y(StartNum+1+5*3).Data  RndMeth=Simplest  InputSameDT=on
  1-D Lookup Table18 : Lookup_n-D  NumberOfTableDimensions=1  BreakpointsForDimension1=TestData_001.X.Data  Table=TestData_001.Y(StartNum+5*3).Data  RndMeth=Simplest  InputSameDT=on
  1-D Lookup Table19 : Lookup_n-D  NumberOfTableDimensions=1  BreakpointsForDimension1=TestData_001.X.Data  Table=TestData_001.Y(StartNum+2+5*3).Data  RndMeth=Simplest  InputSameDT=on
  1-D Lookup Table2 : Lookup_n-D  NumberOfTableDimensions=1  BreakpointsForDimension1=TestData_001.X.Data  Table=TestData_001.Y(StartNum+5*0).Data  RndMeth=Simplest  InputSameDT=on
  1-D Lookup Table20 : Lookup_n-D  NumberOfTableDimensions=1  BreakpointsForDimension1=TestData_001.X.Data  Table=TestData_001.Y(StartNum+3+5*3).Data  RndMeth=Simplest  InputSameDT=on
  1-D Lookup Table21 : Lookup_n-D  NumberOfTableDimensions=1  BreakpointsForDimension1=TestData_001.X.Data  Table=TestData_001.Y(StartNum+4+5*4).Data  RndMeth=Simplest  InputSameDT=on
  1-D Lookup Table22 : Lookup_n-D  NumberOfTableDimensions=1  BreakpointsForDimension1=TestData_001.X.Data  Table=TestData_001.Y(StartNum+1+5*4).Data  RndMeth=Simplest  InputSameDT=on
  1-D Lookup Table23 : Lookup_n-D  NumberOfTableDimensions=1  BreakpointsForDimension1=TestData_001.X.Data  Table=TestData_001.Y(StartNum+5*4).Data  RndMeth=Simplest  InputSameDT=on
  1-D Lookup Table24 : Lookup_n-D  NumberOfTableDimensions=1  BreakpointsForDimension1=TestData_001.X.Data  Table=TestData_001.Y(StartNum+2+5*4).Data  RndMeth=Simplest  InputSameDT=on
  1-D Lookup Table25 : Lookup_n-D  NumberOfTableDimensions=1  BreakpointsForDimension1=TestData_001.X.Data  Table=TestData_001.Y(StartNum+3+5*4).Data  RndMeth=Simplest  InputSameDT=on
  1-D Lookup Table26 : Lookup_n-D  NumberOfTableDimensions=1  BreakpointsForDimension1=TestData_001.X.Data  Table=TestData_001.Y(StartNum+4+5*5).Data  RndMeth=Simplest  InputSameDT=on
  1-D Lookup Table27 : Lookup_n-D  NumberOfTableDimensions=1  BreakpointsForDimension1=TestData_001.X.Data  Table=TestData_001.Y(StartNum+1+5*5).Data  RndMeth=Simplest  InputSameDT=on
  1-D Lookup Table28 : Lookup_n-D  NumberOfTableDimensions=1  BreakpointsForDimension1=TestData_001.X.Data  Table=TestData_001.Y(StartNum+5*5).Data  RndMeth=Simplest  InputSameDT=on
  1-D Lookup Table29 : Lookup_n-D  NumberOfTableDimensions=1  BreakpointsForDimension1=TestData_001.X.Data  Table=TestData_001.Y(StartNum+2+5*5).Data  RndMeth=Simplest  InputSameDT=on
  1-D Lookup Table3 : Lookup_n-D  NumberOfTableDimensions=1  BreakpointsForDimension1=TestData_001.X.Data  Table=TestData_001.Y(StartNum+2+5*0).Data  RndMeth=Simplest  InputSameDT=on
  1-D Lookup Table30 : Lookup_n-D  NumberOfTableDimensions=1  BreakpointsForDimension1=TestData_001.X.Data  Table=TestData_001.Y(StartNum+3+5*5).Data  RndMeth=Simplest  InputSameDT=on
  1-D Lookup Table31 : Lookup_n-D  NumberOfTableDimensions=1  BreakpointsForDimension1=TestData_001.X.Data  Table=TestData_001.Y(StartNum+4+5*6).Data  RndMeth=Simplest  InputSameDT=on
  1-D Lookup Table32 : Lookup_n-D  NumberOfTableDimensions=1  BreakpointsForDimension1=TestData_001.X.Data  Table=TestData_001.Y(StartNum+1+5*6).Data  RndMeth=Simplest  InputSameDT=on
  1-D Lookup Table33 : Lookup_n-D  NumberOfTableDimensions=1  BreakpointsForDimension1=TestData_001.X.Data  Table=TestData_001.Y(StartNum+5*6).Data  RndMeth=Simplest  InputSameDT=on
  1-D Lookup Table34 : Lookup_n-D  NumberOfTableDimensions=1  BreakpointsForDimension1=TestData_001.X.Data  Table=TestData_001.Y(StartNum+2+5*6).Data  RndMeth=Simplest  InputSameDT=on
  1-D Lookup Table35 : Lookup_n-D  NumberOfTableDimensions=1  BreakpointsForDimension1=TestData_001.X.Data  Table=TestData_001.Y(StartNum+3+5*6).Data  RndMeth=Simplest  InputSameDT=on
  1-D Lookup Table36 : Lookup_n-D  NumberOfTableDimensions=1  BreakpointsForDimension1=TestData_001.X.Data  Table=TestData_001.Y(StartNum+4+5*7).Data  RndMeth=Simplest  InputSameDT=on
  1-D Lookup Table37 : Lookup_n-D  NumberOfTableDimensions=1  BreakpointsForDimension1=TestData_001.X.Data  Table=TestData_001.Y(StartNum+1+5*7).Data  RndMeth=Simplest  InputSameDT=on
  1-D Lookup Table38 : Lookup_n-D  NumberOfTableDimensions=1  BreakpointsForDimension1=TestData_001.X.Data  Table=TestData_001.Y(StartNum+5*7).Data  RndMeth=Simplest  InputSameDT=on
  1-D Lookup Table39 : Lookup_n-D  NumberOfTableDimensions=1  BreakpointsForDimension1=TestData_001.X.Data  Table=TestData_001.Y(StartNum+2+5*7).Data  RndMeth=Simplest  InputSameDT=on
  1-D Lookup Table4 : Lookup_n-D  NumberOfTableDimensions=1  BreakpointsForDimension1=TestData_001.X.Data  Table=TestData_001.Y(StartNum+3+5*0).Data  RndMeth=Simplest  InputSameDT=on
  1-D Lookup Table40 : Lookup_n-D  NumberOfTableDimensions=1  BreakpointsForDimension1=TestData_001.X.Data  Table=TestData_001.Y(StartNum+3+5*7).Data  RndMeth=Simplest  InputSameDT=on
  1-D Lookup Table41 : Lookup_n-D  NumberOfTableDimensions=1  BreakpointsForDimension1=TestData_001.X.Data  Table=TestData_001.Y(StartNum+4+5*8).Data  RndMeth=Simplest  InputSameDT=on
  1-D Lookup Table42 : Lookup_n-D  NumberOfTableDimensions=1  BreakpointsForDimension1=TestData_001.X.Data  Table=TestData_001.Y(StartNum+1+5*8).Data  RndMeth=Simplest  InputSameDT=on
  1-D Lookup Table43 : Lookup_n-D  NumberOfTableDimensions=1  BreakpointsForDimension1=TestData_001.X.Data  Table=TestData_001.Y(StartNum+5*8).Data  RndMeth=Simplest  InputSameDT=on
  1-D Lookup Table44 : Lookup_n-D  NumberOfTableDimensions=1  BreakpointsForDimension1=TestData_001.X.Data  Table=TestData_001.Y(StartNum+2+5*8).Data  RndMeth=Simplest  InputSameDT=on
  1-D Lookup Table45 : Lookup_n-D  NumberOfTableDimensions=1  BreakpointsForDimension1=TestData_001.X.Data  Table=TestData_001.Y(StartNum+3+5*8).Data  RndMeth=Simplest  InputSameDT=on
  1-D Lookup Table46 : Lookup_n-D  NumberOfTableDimensions=1  BreakpointsForDimension1=TestData_001.X.Data  Table=TestData_001.Y(StartNum+4+5*9).Data  RndMeth=Simplest  InputSameDT=on
  1-D Lookup Table47 : Lookup_n-D  NumberOfTableDimensions=1  BreakpointsForDimension1=TestData_001.X.Data  Table=TestData_001.Y(StartNum+1+5*9).Data  RndMeth=Simplest  InputSameDT=on
  1-D Lookup Table48 : Lookup_n-D  NumberOfTableDimensions=1  BreakpointsForDimension1=TestData_001.X.Data  Table=TestData_001.Y(StartNum+5*9).Data  RndMeth=Simplest  InputSameDT=on
  1-D Lookup Table49 : Lookup_n-D  NumberOfTableDimensions=1  BreakpointsForDimension1=TestData_001.X.Data  Table=TestData_001.Y(StartNum+2+5*9).Data  RndMeth=Simplest  InputSameDT=on
  1-D Lookup Table5 : Lookup_n-D  NumberOfTableDimensions=1  BreakpointsForDimension1=TestData_001.X.Data  Table=TestData_001.Y(StartNum+4+5*0).Data  RndMeth=Simplest  InputSameDT=on
  1-D Lookup Table50 : Lookup_n-D  NumberOfTableDimensions=1  BreakpointsForDimension1=TestData_001.X.Data  Table=TestData_001.Y(StartNum+3+5*9).Data  RndMeth=Simplest  InputSameDT=on
  1-D Lookup Table6 : Lookup_n-D  NumberOfTableDimensions=1  BreakpointsForDimension1=TestData_001.X.Data  Table=TestData_001.Y(StartNum+1+5*1).Data  RndMeth=Simplest  InputSameDT=on
  1-D Lookup Table7 : Lookup_n-D  NumberOfTableDimensions=1  BreakpointsForDimension1=TestData_001.X.Data  Table=TestData_001.Y(StartNum+5*1).Data  RndMeth=Simplest  InputSameDT=on
  1-D Lookup Table8 : Lookup_n-D  NumberOfTableDimensions=1  BreakpointsForDimension1=TestData_001.X.Data  Table=TestData_001.Y(StartNum+2+5*1).Data  RndMeth=Simplest  InputSameDT=on
  1-D Lookup Table9 : Lookup_n-D  NumberOfTableDimensions=1  BreakpointsForDimension1=TestData_001.X.Data  Table=TestData_001.Y(StartNum+3+5*1).Data  RndMeth=Simplest  InputSameDT=on
  Add : Sum  Inputs=++++++++++
  Constant1 : Constant  Value=[0 1 0 0 0 0 0 0 0 0]
  Constant10 : Constant  Value=[0 0 0 0 0 0 0 0 0 1]
  Constant2 : Constant  Value=[0 0 1 0 0 0 0 0 0 0]
  Constant3 : Constant  Value=[0 0 0 1 0 0 0 0 0 0]
  Constant4 : Constant  Value=[1 0 0 0 0 0 0 0 0 0]
  Constant5 : Constant  Value=[0 0 0 0 1 0 0 0 0 0]
  Constant6 : Constant  Value=[0 0 0 0 0 1 0 0 0 0]
  Constant7 : Constant  Value=[0 0 0 0 0 0 1 0 0 0]
  Constant8 : Constant  Value=[0 0 0 0 0 0 0 1 0 0]
  Constant9 : Constant  Value=[0 0 0 0 0 0 0 0 1 0]
  Divide{,1..9} (10 alike) : Product  Inputs=**  Multiplication=Matrix(*)
  Math Function{,1..10} (11 alike) : Math  Operator=transpose  SaturateOnIntegerOverflow=on
  Mux{1..10} (10 alike) : Mux  Inputs=5
  Quantizer{1..10} (10 alike) : Quantizer  QuantizationInterval=1
  RRSRR[10X5] : Outport
  wires:
  Mux5/1 -> Divide/1
  Constant4/1 -> Math Function/1
  Math Function/1 -> Divide/2
  Divide/1 -> Add/1
  Math Function4/1 -> Divide4/2
  Math Function3/1 -> Divide3/2
  Divide3/1 -> Add/4
  Constant9/1 -> Math Function8/1
  Math Function6/1 -> Divide6/2
  Divide1/1 -> Add/2
  Divide4/1 -> Add/5
  Quantizer9/1 -> Mux5/1
  Constant7/1 -> Math Function6/1
  Divide2/1 -> Add/3
  Divide9/1 -> Add/10
  Constant3/1 -> Math Function3/1
  Divide5/1 -> Add/6
  Math Function5/1 -> Divide5/2
  1-D Lookup Table4/1 -> Mux5/4
  1-D Lookup Table3/1 -> Mux5/3
  Constant8/1 -> Math Function7/1
  Divide6/1 -> Add/7
  Math Function8/1 -> Divide8/2
  Constant5/1 -> Math Function4/1
  Math Function9/1 -> Divide9/2
  Math Function7/1 -> Divide7/2
  Constant10/1 -> Math Function9/1
  Math Function2/1 -> Divide2/2
  Constant1/1 -> Math Function1/1
  Divide7/1 -> Add/8
  Divide8/1 -> Add/9
  Constant2/1 -> Math Function2/1
  Math Function1/1 -> Divide1/2
  Constant6/1 -> Math Function5/1
  Add/1 -> Math Function10/1
  Math Function10/1 -> RRSRR[10X5]/1
  1-D Lookup Table2/1 -> Quantizer9/1
  [Clock] -> 1-D Lookup Table2/1, 1-D Lookup Table1/1, 1-D Lookup Table5/1, 1-D Lookup Table4/1, 1-D Lookup Table3/1
  1-D Lookup Table1/1 -> Mux5/2  "Data"
  1-D Lookup Table5/1 -> Mux5/5
  Mux1/1 -> Divide1/1
  Quantizer1/1 -> Mux1/1
  1-D Lookup Table9/1 -> Mux1/4
  1-D Lookup Table8/1 -> Mux1/3
  1-D Lookup Table7/1 -> Quantizer1/1
  [Clock] -> 1-D Lookup Table7/1, 1-D Lookup Table6/1, 1-D Lookup Table8/1, 1-D Lookup Table10/1, 1-D Lookup Table9/1
  1-D Lookup Table6/1 -> Mux1/2  "Data"
  1-D Lookup Table10/1 -> Mux1/5
  Mux2/1 -> Divide2/1
  Quantizer2/1 -> Mux2/1
  1-D Lookup Table15/1 -> Mux2/4
  1-D Lookup Table14/1 -> Mux2/3
  1-D Lookup Table13/1 -> Quantizer2/1
  [Clock] -> 1-D Lookup Table13/1, 1-D Lookup Table12/1, 1-D Lookup Table14/1, 1-D Lookup Table15/1, 1-D Lookup Table11/1
  1-D Lookup Table12/1 -> Mux2/2  "Data"
  1-D Lookup Table11/1 -> Mux2/5
  Mux3/1 -> Divide3/1
  Quantizer3/1 -> Mux3/1
  1-D Lookup Table20/1 -> Mux3/4
  1-D Lookup Table19/1 -> Mux3/3
  1-D Lookup Table18/1 -> Quantizer3/1
  [Clock] -> 1-D Lookup Table18/1, 1-D Lookup Table17/1, 1-D Lookup Table19/1, 1-D Lookup Table20/1, 1-D Lookup Table16/1
  1-D Lookup Table17/1 -> Mux3/2  "Data"
  1-D Lookup Table16/1 -> Mux3/5
  Mux4/1 -> Divide4/1
  Quantizer4/1 -> Mux4/1
  1-D Lookup Table25/1 -> Mux4/4
  1-D Lookup Table24/1 -> Mux4/3
  1-D Lookup Table23/1 -> Quantizer4/1
  [Clock] -> 1-D Lookup Table23/1, 1-D Lookup Table22/1, 1-D Lookup Table24/1, 1-D Lookup Table21/1, 1-D Lookup Table25/1
  1-D Lookup Table22/1 -> Mux4/2  "Data"
  1-D Lookup Table21/1 -> Mux4/5
  Mux6/1 -> Divide5/1
  Quantizer5/1 -> Mux6/1
  1-D Lookup Table30/1 -> Mux6/4
  1-D Lookup Table29/1 -> Mux6/3
  1-D Lookup Table28/1 -> Quantizer5/1
  [Clock] -> 1-D Lookup Table28/1, 1-D Lookup Table27/1, 1-D Lookup Table29/1, 1-D Lookup Table30/1, 1-D Lookup Table26/1
  1-D Lookup Table27/1 -> Mux6/2  "Data"
  1-D Lookup Table26/1 -> Mux6/5
  Mux7/1 -> Divide6/1
  Quantizer6/1 -> Mux7/1
  1-D Lookup Table35/1 -> Mux7/4
  1-D Lookup Table34/1 -> Mux7/3
  1-D Lookup Table33/1 -> Quantizer6/1
  [Clock] -> 1-D Lookup Table33/1, 1-D Lookup Table32/1, 1-D Lookup Table34/1, 1-D Lookup Table31/1, 1-D Lookup Table35/1
  1-D Lookup Table32/1 -> Mux7/2  "Data"
  1-D Lookup Table31/1 -> Mux7/5
  Mux8/1 -> Divide7/1
  Quantizer7/1 -> Mux8/1
  1-D Lookup Table40/1 -> Mux8/4
  1-D Lookup Table39/1 -> Mux8/3
  1-D Lookup Table38/1 -> Quantizer7/1
  [Clock] -> 1-D Lookup Table38/1, 1-D Lookup Table37/1, 1-D Lookup Table39/1, 1-D Lookup Table40/1, 1-D Lookup Table36/1
  1-D Lookup Table37/1 -> Mux8/2  "Data"
  1-D Lookup Table36/1 -> Mux8/5
  Mux9/1 -> Divide8/1
  Quantizer8/1 -> Mux9/1
  1-D Lookup Table45/1 -> Mux9/4
  1-D Lookup Table44/1 -> Mux9/3
  1-D Lookup Table43/1 -> Quantizer8/1
  [Clock] -> 1-D Lookup Table43/1, 1-D Lookup Table42/1, 1-D Lookup Table44/1, 1-D Lookup Table41/1, 1-D Lookup Table45/1
  1-D Lookup Table42/1 -> Mux9/2  "Data"
  1-D Lookup Table41/1 -> Mux9/5
  Mux10/1 -> Divide9/1
  Quantizer10/1 -> Mux10/1
  1-D Lookup Table50/1 -> Mux10/4
  1-D Lookup Table49/1 -> Mux10/3
  1-D Lookup Table48/1 -> Quantizer10/1
  [Clock] -> 1-D Lookup Table48/1, 1-D Lookup Table47/1, 1-D Lookup Table49/1, 1-D Lookup Table50/1, 1-D Lookup Table46/1
  1-D Lookup Table47/1 -> Mux10/2  "Data"
  1-D Lookup Table46/1 -> Mux10/5

== system ADU_Integration_R2014a_simulation/LogData/Sensor_ESR/Data_1 ==
  1-D Lookup Table1 : Lookup_n-D  NumberOfTableDimensions=1  BreakpointsForDimension1=TestData_001.X.Data  Table=TestData_001.Y(206+4*a).Data  RndMeth=Simplest  InputSameDT=on
  1-D Lookup Table2 : Lookup_n-D  NumberOfTableDimensions=1  BreakpointsForDimension1=TestData_001.X.Data  Table=TestData_001.Y(205+4*a).Data  RndMeth=Simplest  InputSameDT=on
  1-D Lookup Table3 : Lookup_n-D  NumberOfTableDimensions=1  BreakpointsForDimension1=TestData_001.X.Data  Table=TestData_001.Y(207+4*a).Data  RndMeth=Simplest  InputSameDT=on
  1-D Lookup Table4 : Lookup_n-D  NumberOfTableDimensions=1  BreakpointsForDimension1=TestData_001.X.Data  Table=TestData_001.Y(208+4*a).Data  RndMeth=Simplest  InputSameDT=on
  Mux5 : Mux
  Quantizer9 : Quantizer  QuantizationInterval=1
  Out1 : Outport
  wires:
  Mux5/1 -> Out1/1
  [Clock] -> 1-D Lookup Table2/1, 1-D Lookup Table4/1, 1-D Lookup Table3/1, 1-D Lookup Table1/1
  1-D Lookup Table4/1 -> Mux5/4
  Quantizer9/1 -> Mux5/1
  1-D Lookup Table2/1 -> Quantizer9/1
  1-D Lookup Table1/1 -> Mux5/2  "Data"
  1-D Lookup Table3/1 -> Mux5/3

== system ADU_Integration_R2014a_simulation/LogData/Sensor_ESR/Data_10 ==
  1-D Lookup Table1 : Lookup_n-D  NumberOfTableDimensions=1  BreakpointsForDimension1=TestData_001.X.Data  Table=TestData_001.Y(206+4*a).Data  RndMeth=Simplest  InputSameDT=on
  1-D Lookup Table2 : Lookup_n-D  NumberOfTableDimensions=1  BreakpointsForDimension1=TestData_001.X.Data  Table=TestData_001.Y(205+4*a).Data  RndMeth=Simplest  InputSameDT=on
  1-D Lookup Table3 : Lookup_n-D  NumberOfTableDimensions=1  BreakpointsForDimension1=TestData_001.X.Data  Table=TestData_001.Y(207+4*a).Data  RndMeth=Simplest  InputSameDT=on
  1-D Lookup Table4 : Lookup_n-D  NumberOfTableDimensions=1  BreakpointsForDimension1=TestData_001.X.Data  Table=TestData_001.Y(208+4*a).Data  RndMeth=Simplest  InputSameDT=on
  Mux5 : Mux
  Quantizer9 : Quantizer  QuantizationInterval=1
  Out1 : Outport
  wires:
  1-D Lookup Table3/1 -> Mux5/3
  1-D Lookup Table1/1 -> Mux5/2  "Data"
  1-D Lookup Table2/1 -> Quantizer9/1
  Quantizer9/1 -> Mux5/1
  1-D Lookup Table4/1 -> Mux5/4
  [Clock] -> 1-D Lookup Table1/1, 1-D Lookup Table3/1, 1-D Lookup Table4/1, 1-D Lookup Table2/1
  Mux5/1 -> Out1/1

== system ADU_Integration_R2014a_simulation/LogData/Sensor_ESR/Data_11 ==
  1-D Lookup Table1 : Lookup_n-D  NumberOfTableDimensions=1  BreakpointsForDimension1=TestData_001.X.Data  Table=TestData_001.Y(206+4*a).Data  RndMeth=Simplest  InputSameDT=on
  1-D Lookup Table2 : Lookup_n-D  NumberOfTableDimensions=1  BreakpointsForDimension1=TestData_001.X.Data  Table=TestData_001.Y(205+4*a).Data  RndMeth=Simplest  InputSameDT=on
  1-D Lookup Table3 : Lookup_n-D  NumberOfTableDimensions=1  BreakpointsForDimension1=TestData_001.X.Data  Table=TestData_001.Y(207+4*a).Data  RndMeth=Simplest  InputSameDT=on
  1-D Lookup Table4 : Lookup_n-D  NumberOfTableDimensions=1  BreakpointsForDimension1=TestData_001.X.Data  Table=TestData_001.Y(208+4*a).Data  RndMeth=Simplest  InputSameDT=on
  Mux5 : Mux
  Quantizer9 : Quantizer  QuantizationInterval=1
  Out1 : Outport
  wires:
  Mux5/1 -> Out1/1
  [Clock] -> 1-D Lookup Table2/1, 1-D Lookup Table4/1, 1-D Lookup Table3/1, 1-D Lookup Table1/1
  1-D Lookup Table4/1 -> Mux5/4
  Quantizer9/1 -> Mux5/1
  1-D Lookup Table2/1 -> Quantizer9/1
  1-D Lookup Table1/1 -> Mux5/2  "Data"
  1-D Lookup Table3/1 -> Mux5/3

== system ADU_Integration_R2014a_simulation/LogData/Sensor_ESR/Data_12 ==
  1-D Lookup Table1 : Lookup_n-D  NumberOfTableDimensions=1  BreakpointsForDimension1=TestData_001.X.Data  Table=TestData_001.Y(206+4*a).Data  RndMeth=Simplest  InputSameDT=on
  1-D Lookup Table2 : Lookup_n-D  NumberOfTableDimensions=1  BreakpointsForDimension1=TestData_001.X.Data  Table=TestData_001.Y(205+4*a).Data  RndMeth=Simplest  InputSameDT=on
  1-D Lookup Table3 : Lookup_n-D  NumberOfTableDimensions=1  BreakpointsForDimension1=TestData_001.X.Data  Table=TestData_001.Y(207+4*a).Data  RndMeth=Simplest  InputSameDT=on
  1-D Lookup Table4 : Lookup_n-D  NumberOfTableDimensions=1  BreakpointsForDimension1=TestData_001.X.Data  Table=TestData_001.Y(208+4*a).Data  RndMeth=Simplest  InputSameDT=on
  Mux5 : Mux
  Quantizer9 : Quantizer  QuantizationInterval=1
  Out1 : Outport
  wires:
  1-D Lookup Table3/1 -> Mux5/3
  1-D Lookup Table1/1 -> Mux5/2  "Data"
  1-D Lookup Table2/1 -> Quantizer9/1
  Quantizer9/1 -> Mux5/1
  1-D Lookup Table4/1 -> Mux5/4
  [Clock] -> 1-D Lookup Table1/1, 1-D Lookup Table3/1, 1-D Lookup Table4/1, 1-D Lookup Table2/1
  Mux5/1 -> Out1/1
